simulink model "IEEE9-WT-PV"  (R2024a)
settings: Solver=FixedStepDiscrete  StartTime=0.0  StopTime=Tend  RelTol=1e-3
values from neighbouring files (symbols this model uses):
  beta_0 = 0    [data_WT.m]
  C_4 = 0.1670*C_b    (= 1.00487241952e-06)    [main.m]
  C_6 = 0.2835*C_b    (= 1.70587623314e-06)    [main.m]
  C_8 = 0.2275*C_b    (= 1.36891302659e-06)    [main.m]
  C_dc = 2*S_LV_base*H_DC_base/V_dc_base^2    (= 0.478267523722)    [data_WT.m]    (also in main.m = 1.6)
  C_f = C_f_pu*C_LV_base    (= 0.001461477898)    [data_WT.m]    (also in main.m = 0.00530516476973)
  f_b = 50    [data_WT.m]    (also in main.m)
  fdr_m = 0.05    [main.m]
  fdr_q = 0.01    [main.m]
  G_diff = ss(c2d(s/(20e-3/3*s+1),T_s_cont,'tustin'))    [data_WT.m]
  G_lowpass_disc = ss(c2d(G_lowpass,T_s_cont,'tustin'))    [data_WT.m]
  G_lowpass_disc_1khz = ss(c2d(G_lowpass_1khz,T_s_cont,'tustin'))    [data_WT.m]
  G_setpoint_lowpass_disc = ss(c2d(ss(1/(0.1*s+1)),T_s_cont,'tustin'))    [main.m]
  G_sm_dis = ss(c2d(G_cont_sm,T_s_sim,'tustin'))    [main.m]
  GSC_theta0 = -45.0572/180*pi*0-60/180*pi    (= -1.0471975512)    [data_WT.m]
  I0_total1 = Npar1*I0    (= 7.7895e-08)    [data_PV.m]
  I_GSC_base = S_GSC_base/V_LV_base    (= 30303.030303)    [data_WT.m]
  I_PMSG_0 = T_park(0)^-1*[Z_PMSG^-1*V_LV_base*sqrt(2/3)*([cos(RSC_theta0);sin(RSC_theta0)]-[cos(PMSG_theta0);sin(PMSG_theta0)]);0]    [data_WT.m]
  IL_total1 = Npar1*IL    (= 50459)    [data_PV.m]
  Ipv_scmax1 = Npar1*Ipv_sc    (= 50300)    [data_PV.m]
  island_q = [-0.1312   -0.0230   -0.0343]    [main.m]
  island_Vdc = [1 1.2853    Vpv_mppmax2/Vdc_n]    [main.m]
  island_Vdc_r = [1 1.3430 1.4716]    [main.m]
  island_Vm = [1 1 1]    [main.m]
  J_PMSG_WT_MS = 2*H_PMSGWT_LS*S_PMSG_base/(2*pi*f_b)^2    (= 630.526507942)    [data_WT.m]
  k_p_GSC = 0.02    [data_WT.m]
  k_p_MSC = k_p_GSC    (= 0.02)    [data_WT.m]
  k_theta_GSC = 0.1    [data_WT.m]
  k_theta_MSC = 2/0.6    (= 3.33333333333)    [data_WT.m]
  K_WT_ff_i = 1    [main.m]
  K_WT_ff_v = 1    [main.m]
  K_WT_i_i = 0.79    [main.m]
  K_WT_i_v = 0.69    [main.m]
  K_WT_p_i = 2.1    [main.m]
  K_WT_p_v = 0.15    [main.m]
  Kff_v = 1    [main.m]
  Kffpv_i = 1    [main.m]
  Kp_beta = 270*0    (= 0)    [data_WT.m]
  Kpvi_i1 = Ki_i*Vpv_m/Ipv_b_LV    [main.m]
  Kpvi_v1 = Ki_v*Ipv_b_LV/Vpv_m    [main.m]
  Kpvp_i1 = Kp_i*Vpv_m/Ipv_b_LV    [main.m]
  Kpvp_v1 = Kp_v*Ipv_b_LV/Vpv_m    [main.m]
  L1_pu = 1*0.0186/m    (= 0.000186)    [main.m]
  L_45 = L_lines(2)    [main.m]
  L_56 = L_lines(3)    [main.m]
  L_67 = L_lines(5)    [main.m]
  L_78 = L_lines(6)    [main.m]
  L_89 = L_lines(8)    [main.m]
  L_94 = L_lines(9)    [main.m]
  L_f = L_f_pu*L_LV_base    (= 3.46639466054e-05)    [data_WT.m]    (also in main.m = 9.54929658551e-06)
  L_PMSG = L_PMSG_PU*L_LV_base    (= 3.46639466054e-05)    [data_WT.m]
  main_p = 0.575    [main.m]
  mpv_dc1 = fdr*kg1*w_b/Vdc_n    [main.m]
  mpv_dc1_r = fdr*kg1_r*w_b/Vdc_n    [main.m]
  mpv_p1 = fdr_p/Vdc_n*w_b    [main.m]
  mpv_q1 = fdr_q*Vpv_m/S_b    [main.m]
  Notch_w_10khz = ss(c2d((s^2+w0_f10khz^2)/(s^2+w0_f10khz/Q_f10khz*s+w0_f10khz^2),T_s_sim,'tustin'))    [data_WT.m]
  omega_base = 2*pi*f_b    (= 314.159265359)    [data_WT.m]    (also in main.m)
  omega_wt = 1.4    [data_WT.m]
  R1_pu = 1*0.00734/m    (= 7.34e-05)    [main.m]
  R_45 = R_lines(2)    [main.m]
  R_56 = R_lines(3)    [main.m]
  R_67 = R_lines(5)    [main.m]
  R_78 = R_lines(6)    [main.m]
  R_89 = R_lines(8)    [main.m]
  R_94 = R_lines(9)    [main.m]
  R_f = R_f_pu*Z_LV_base    (= 0.001089)    [data_WT.m]    (also in main.m = 0.0003)
  R_PMSG = R_PMSG_PU*Z_LV_base    (= 0.005445)    [data_WT.m]
  Rpvs_total1 = Rpv_s*Nser1/Npar1    (= 0.0067482)    [data_PV.m]
  RSC_theta0 = 180/180*pi    (= 3.14159265359)    [data_WT.m]
  Rss1 = Vpv_ocmax1/(IL_total1-I0_total1*(exp(Vpv_ocmax1/VT_total1) -1))    [data_PV.m]
  S_b = 100*(10^6)    (= 100000000)    [main.m]
  S_bt = S_b    (= 100000000)    [main.m]
  S_GSC_base = S_LV_base    (= 100000000)    [data_WT.m]
  S_PMSG_base = S_WTPMSG_base    (= 100000000)    [data_WT.m]
  T_load = 20    [main.m]
  T_pitch_servo = 0.5    [data_WT.m]
  T_redispatch = 25    [main.m]
  T_s_cont = 1e-4    (= 0.0001)    [data_WT.m]
  T_s_sim = 1e-7    (= 1e-07)    [data_WT.m]
  V1_rms = 1000    [main.m]
  V2_rms = 13800    [main.m]
  V_dc_base = 7.92e3    (= 7920)    [data_WT.m]
  V_LV_base = 3.3e3    (= 3300)    [data_WT.m]
  V_m = sqrt(2/3)*V1_rms    [main.m]
  v_wind = 12    [data_WT.m]
  Vdc_n = 3*V_m    [main.m]
  Vpv_mppmax1 = Nser1*Vpv_mpp    (= 2945.7)    [data_PV.m]
  Vpv_ocmax1 = Nser1*Vpv_oc    (= 3671.1)    [data_PV.m]
  VT_total1 = VT*Nser1    (= 135.150894483)    [data_PV.m]
  w_b = 2*pi*f_b    (= 314.159265359)    [data_WT.m]    (also in main.m)
undefined symbols (not defined in the file or in its folder): D1, Delta, DiscIntNeverNeededParam, i_dc, PI_pitch
libraries: spsThreePhaseVIMeasurementLib x15, spsThreePhaseSeriesRLCBranchLib x11, spsabctodq0Lib x8, spsThreePhaseTransformerTwoWindingsLib x5, spsThreePhaseParallelRLCLoadLib x5, spsGroundLib x5, spsSeriesRLCBranchLib x5, spsCurrentMeasurementLib x5, spsVoltageMeasurementLib x4, spsPower3phInstantaneousLib x4, spsdq0toabcLib x4, spsThreePhaseParallelRLCBranchLib x3
(part 2 of 3)

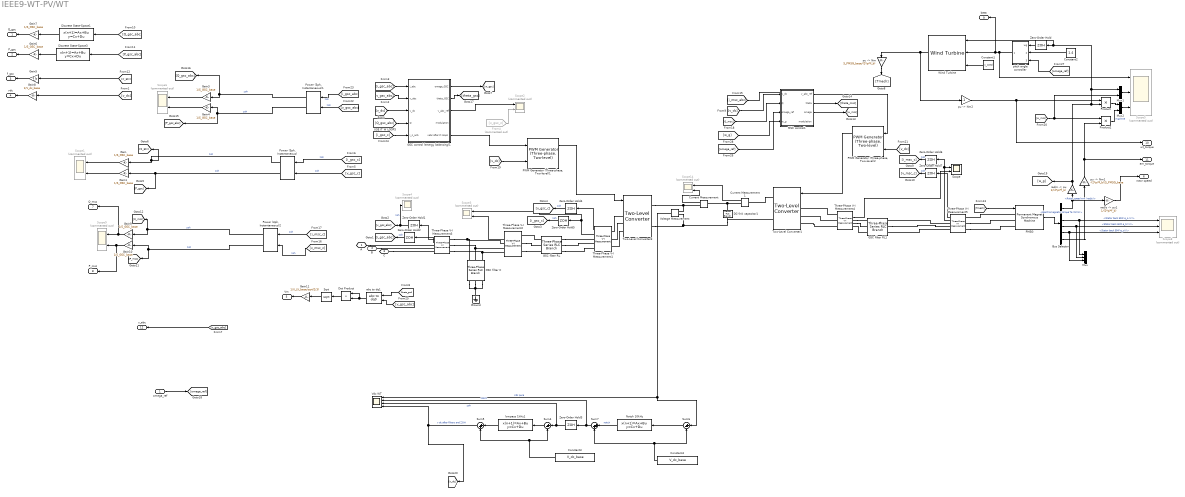
== system IEEE9-WT-PV/WT ==
  omega_ref : Inport
  Bus Selector : BusSelector  OutputSignals=Rotor speed wm (rad/s),Rotor angle thetam (rad),Stator back EMF e_a (V),Stator back EMF e_b (V),Stator back EMF e_cV),Electromagnetic torque Te (N*m)
  Constant1 : Constant  Value=v_wind  SampleTime=T_s_sim
  Constant2 : Constant  Value=1.4  SampleTime=T_s_cont
  Constant3 : Constant  Value=V_dc_base  SampleTime=T_s_cont
  Constant4 : Constant  Value=V_dc_base  SampleTime=T_s_sim
  Current Measurement : spsCurrentMeasurementLib/Current Measurement  PhasorSimulation=off  OutputType=Complex  PSBequivalent=0
  Current Measurement1 : spsCurrentMeasurementLib/Current Measurement  PhasorSimulation=off  OutputType=Complex  PSBequivalent=0
  DC-link capacitor1 : spsSeriesRLCBranchLib/Series RLC Branch  LConnTagsString=__new0  RConnTagsString=__new0  BranchType=C  Resistance=1  Inductance=1e-3  SetiL0=off  InitialCurrent=0  Capacitance=C_dc  Setx0=on  InitialVoltage=V_dc_base  Measurements=None
  Discrete State-Space1 : DiscreteStateSpace  A=G_lowpass_disc.A  B=G_lowpass_disc.B  C=G_lowpass_disc.C  D=G_lowpass_disc.D  SampleTime=T_s_cont
  Discrete State-Space3 : DiscreteStateSpace  A=G_lowpass_disc.A  B=G_lowpass_disc.B  C=G_lowpass_disc.C  D=G_lowpass_disc.D  SampleTime=T_s_cont
  Dot Product : DotProduct  OutDataTypeStr=Inherit: Inherit via internal rule
  From4 : From  Commented=on  GotoTag=v_gsc_c
  GSC control (energy balancing)1 : Subsystem
  GSC filter C : spsThreePhaseSeriesRLCBranchLib/Three-Phase Series RLC Branch  LConnTagsString=A|B|C  RConnTagsString=A|B|C  BranchType=C  Resistance=R_f  Inductance=L_f  Capacitance=C_f  Measurements=None
  GSC filter RL : spsThreePhaseSeriesRLCBranchLib/Three-Phase Series RLC Branch  LConnTagsString=A|B|C  RConnTagsString=A|B|C  BranchType=RL  Resistance=R_f  Inductance=L_f  Capacitance=1e-6  Measurements=None
  GSC filter RL1 : spsThreePhaseSeriesRLCBranchLib/Three-Phase Series RLC Branch  LConnTagsString=A|B|C  RConnTagsString=A|B|C  BranchType=RL  Resistance=R_f  Inductance=L_f  Capacitance=1e-6  Measurements=None
  Gain{,1,3..4,6..7,9..10} (8 alike) : Gain  Gain=1/S_GSC_base
  Gain11 : Gain  Gain=1/V_LV_base/sqrt(2/3)
  Gain5 : Gain  Gain=f_b
  Gain8 : Gain  Gain=1/V_dc_base
  Ground : spsGroundLib/Ground  LConnTagsString=a
  MSC control1 : Subsystem
  Mux : Mux  Inputs=3
  Mux1 : Mux  Inputs=2
  Mux2 : Mux  Inputs=2
  Notch 10kHz : DiscreteStateSpace  A=Notch_w_10khz.A  B=Notch_w_10khz.B  C=Notch_w_10khz.C  D=Notch_w_10khz.D  SampleTime=T_s_sim
  PMSG : spsPermanentMagnetSynchronousMachineLib/Permanent Magnet Synchronous Machine  NbPhases=3  FluxDistribution=Trapezoidal  RotorType=Round  MechanicalLoad=Torque Tm  PresetModel=No  ShowDetailedParameters=on  MeasurementBus=off  Resistance=R_PMSG  Inductance=L_PMSG  dqInductances=[8.5e-3,8.5e-3]  La=L_PMSG  MachineConstant=Flux linkage established by magnets (V.s)  Flux=V_LV_base/(omega_wt*f_b*2*pi)*sqrt(2/3)*1  VoltageCst=1111.1678  TorqueCst=10.6109  Flat=0  Mechanical=[J_PMSG_WT_MS 0.001 1 0]  PolePairs=1  InitialConditions=[omega_wt*f_b*2*pi,0, I_PMSG_0(1),I_PMSG_0(2)]  InitialConditions5ph=[0 0 0 0 0 0]  RefAngle=Aligned with phase A axis (original Park)  IterativeDiscreteModel=Backward Euler robust  TsBlock=T_s_sim  TsPowergui=0
  "PWM Generator (Three-phase, Two-level)1" : eePwmGeneratorTwoLevel/PWM Generator (Three-phase, Two-level)  PWMMode=Continuous PWM (CPWM)  CPWMMode=SPWM: sinusoidal PWM  DPWMMode=60 DPWM: 60 degree discontinuous PWM  fsw=10e3  Ts=T_s_sim
  "PWM Generator (Three-phase, Two-level)2" : eePwmGeneratorTwoLevel/PWM Generator (Three-phase, Two-level)  PWMMode=Continuous PWM (CPWM)  CPWMMode=SPWM: sinusoidal PWM  DPWMMode=60 DPWM: 60 degree discontinuous PWM  fsw=10e3  Ts=T_s_sim
  "Power (3ph, Instantaneous)" : spsPower3phInstantaneousLib/Power (3ph, Instantaneous)
  "Power (3ph, Instantaneous)1" : spsPower3phInstantaneousLib/Power (3ph, Instantaneous)
  "Power (3ph, Instantaneous)2" : spsPower3phInstantaneousLib/Power (3ph, Instantaneous)
  Product : Product
  Product1 : Product
  Scope : Scope  NumInputPorts=2
  Scope{1..3,6,9,14} (6 alike) : Scope  Commented=on  NumInputPorts=2
  Scope4 : Scope  Commented=on
  Scope5 : Scope  Commented=on  NumInputPorts=3
  Scope8 : Scope  Commented=on  NumInputPorts=3
  Sqrt : Sqrt
  Sum4 : Sum  Inputs=|+-
  Sum5 : Sum  Inputs=|++
  Sum6 : Sum  Inputs=|+-
  Sum7 : Sum  Inputs=|++
  Three-Phase V-I Measurement{1..5} (5 alike) : spsThreePhaseVIMeasurementLib/Three-Phase V-I Measurement  VoltageMeasurement=phase-to-ground  SetLabelV=off  LabelV=Vabc  Vpu=off  VpuLL=off  CurrentMeasurement=yes  SetLabelI=off  LabelI=Iabc  Ipu=off  Pbase=100e6  Vbase=500e3  OutputType=Complex  PhasorSimulation=off  PSBequivalent=0
  Two-Level Converter1 : spsTwoLevelConverterLib/Two-Level Converter  ModelType=Switching devices  Ron=1e-3  Rs=1e6  Cs=inf  Vforward=[0,0]  Ron_Diode=1e-3  Rs_Diode=1e6  Cs_Diode=inf  Vf_Diode=1e-3  Rs_CurrentSource=inf  Ron_ACsource=1e-3
  Two-Level Converter3 : spsTwoLevelConverterLib/Two-Level Converter  ModelType=Switching devices  Ron=1e-3  Rs=1e6  Cs=inf  Vforward=[0,0]  Ron_Diode=1e-3  Rs_Diode=1e6  Cs_Diode=inf  Vf_Diode=1e-3  Rs_CurrentSource=inf  Ron_ACsource=1e-3
  Vdc WT : Scope  NumInputPorts=4
  Voltage Measurement : spsVoltageMeasurementLib/Voltage Measurement  PhasorSimulation=off  OutputType=Complex  PSBequivalent=0
  Wind Turbine : spsWindTurbineLib/Wind Turbine  Pnom=S_PMSG_base  Pelec_base=S_PMSG_base  wind_base=12  P_wind_base=0.75  speed_nom=1.2  pitch_angle=beta_0  c1_c6="[0.51763          116          0.4            5           21     0.006795]"  cp_nom=0.48  lambda_nom=8.1
  Zero-Order Hold{,1..7} (8 alike) : ZeroOrderHold  SampleTime=T_s_cont
  abc to dq1 : spsabctodq0Lib/abc to dq0  Alignment=90 degrees behind phase A axis
  lowpass 1kHz1 : DiscreteStateSpace  A=G_lowpass_disc_1khz.A  B=G_lowpass_disc_1khz.B  C=G_lowpass_disc_1khz.C  D=G_lowpass_disc_1khz.D  SampleTime=T_s_cont
  pitch angle controller : Subsystem
  "pu -> Nm" : Gain  Gain=S_PMSG_base/(2*pi*f_b)
  "pu -> Nm1" : Gain  Gain=-(2*pi*f_b)/S_PMSG_base
  "pu -> Nm2" : Gain  Gain=-1
  "rad/s -> pu" : Gain  Gain=1/(2*pi*f_b)
  "rad/s -> pu1" : Gain  Gain=1/(2*pi*f_b)
  A : PMIOPort  Side=Right
  B : PMIOPort  Port=2  Side=Right
  C : PMIOPort  Port=3  Side=Right
  Q_gsc : Outport
  P_gsc : Outport  Port=2
  f_gsc : Outport  Port=3
  vdc : Outport  Port=4
  Vm : Outport  Port=5
  rotor speed : Outport  Port=6
  Q_msc : Outport  Port=7
  P_msc : Outport  Port=8
  beta : Outport  Port=9
  wt_torque : Outport  Port=10
  em_torque : Outport  Port=11
  v_abc : Outport  Port=12  VectorParamsAs1DForOutWhenUnconnected=off
  wires:
  Wind Turbine/1 -> "pu -> Nm"/1, "pu -> Nm2"/1
  "rad/s -> pu"/1 -> Wind Turbine/1, Zero-Order Hold/1, Mux1/1, Product/2, [w_g]
  Constant1/1 -> Wind Turbine/3
  GSC control (energy balancing)1/3(v_abc_ref) -> Scope2/1
  Bus Selector/1 -> "rad/s -> pu1"/1, "rad/s -> pu"/1  "<Rotor speed wm (rad/s)>"
  GSC control (energy balancing)1/1(omega_GSC) -> [w_gsc]
  Bus Selector/4 -> Mux/2, Scope8/2  "<Stator back EMF e_b (V)>"
  Bus Selector/3 -> Mux/1, Scope8/1  "<Stator back EMF e_a (V)>"
  Bus Selector/5 -> Mux/3, Scope8/3  "<Stator back EMF e_cV)>"
  Gain1/1 -> Scope1/2
  Gain/1 -> Scope1/1
  PMSG/1 -> Bus Selector/1
  Constant2/1 -> pitch angle controller/2(max)
  pitch angle controller/1(pitch) -> Scope5/1, Wind Turbine/2, beta/1
  Mux1/1 -> Scope5/2
  Mux2/1 -> Scope5/3
  Product/1 -> Mux2/1
  Bus Selector/6 -> "pu -> Nm1"/1  "<Electromagnetic torque Te (N*m)>"
  Product1/1 -> Mux2/2  "machine"
  "pu -> Nm1"/1 -> em_torque/1, Product1/2
  Gain5/1 -> f_gsc/1
  [v_dc] -> GSC control (energy balancing)1/3(v_dc)
  [v_dc] -> Gain8/1
  Three-Phase V-I Measurement3/1 -> Zero-Order Hold1/1
  [v_gsc_abc] -> GSC control (energy balancing)1/2(v_abc)
  [i_gsc_abc] -> GSC control (energy balancing)1/1(i_abc)
  Three-Phase V-I Measurement1/2 -> Scope3/1, Zero-Order Hold5/1
  Three-Phase V-I Measurement1/1 -> Zero-Order Hold4/1
  From4/1 -> Scope2/2
  [v_dc] -> MSC control1/1(v_dc)
  [Q_gsc_abc] -> Discrete State-Space1/1
  [P_gsc_abc] -> Discrete State-Space3/1
  Gain6/1 -> P_gsc/1
  Gain7/1 -> Q_gsc/1
  Gain8/1 -> vdc/1
  [w_gsc] -> Gain5/1
  "pu -> Nm"/1 -> [Tmech]
  [Tmech] -> PMSG/1
  [i_msc_abc] -> ?
  Gain9/1 -> Q_msc/1, Scope9/1
  Gain10/1 -> P_msc/1, Scope9/2
  MSC control1/3(omega) -> [w_msc]
  [w_msc] -> Mux1/2, Product1/1
  MSC control1/2(theta) -> [theta_msc]
  Gain4/1 -> Scope6/2
  Gain3/1 -> Scope6/1
  Three-Phase V-I Measurement3/2 -> Zero-Order Hold2/1
  Zero-Order Hold/1 -> pitch angle controller/1(wg)
  [i_gsc_c] -> GSC control (energy balancing)1/5(i_s_acb)
  [Q_gsc_abc] -> GSC control (energy balancing)1/4(Q)
  GSC control (energy balancing)1/2(theta_GSC) -> [theta_gsc]
  Current Measurement1/1 -> Scope14/1
  Current Measurement/1 -> Scope14/2
  [theta_gsc] -> abc to dq1/2
  [v_gsc_abc] -> abc to dq1/1
  abc to dq1/1 -> Dot Product/1, Dot Product/2
  Dot Product/1 -> Sqrt/1
  Gain11/1 -> Vm/1
  Sqrt/1 -> Gain11/1
  "rad/s -> pu1"/1 -> rotor speed/1
  "pu -> Nm2"/1 -> wt_torque/1, Product/1
  omega_ref/1 -> [omega_ref]
  [omega_ref] -> MSC control1/3(omega_ref)
  [omega_ref] -> pitch angle controller/3(omega_ref)
  [w_g] -> MSC control1/4(w_g)
  [Q_msc] -> MSC control1/2(Q)
  Three-Phase V-I Measurement5/2 -> Zero-Order Hold6/1, Scope/1
  Constant4/1 -> Sum6/2, Sum7/2
  Notch 10kHz/1 -> Sum7/1  "notch"
  Voltage Measurement/1 -> Sum6/1, Vdc WT/1  "Vdc pure"
  Sum4/1 -> lowpass 1kHz1/1
  lowpass 1kHz1/1 -> Sum5/1
  Sum7/1 -> Zero-Order Hold3/1, Vdc WT/2  "notch"
  Sum6/1 -> Notch 10kHz/1
  Constant3/1 -> Sum4/2, Sum5/2
  GSC control (energy balancing)1/5(vabc after PI loops) -> "PWM Generator (Three-phase, Two-level)1"/1
  [v_dc] -> "PWM Generator (Three-phase, Two-level)1"/2
  [v_dc] -> "PWM Generator (Three-phase, Two-level)2"/2
  [i_msc_c] -> "Power (3ph, Instantaneous)2"/2  "zoh"
  [v_msc_c] -> "Power (3ph, Instantaneous)2"/1  "zoh"
  [v_gsc_c] -> "Power (3ph, Instantaneous)"/1  "zoh"
  [i_gsc_c] -> "Power (3ph, Instantaneous)"/2  "zoh"
  [v_gsc_abc] -> "Power (3ph, Instantaneous)1"/1  "zoh"
  [i_gsc_abc] -> "Power (3ph, Instantaneous)1"/2  "zoh"
  MSC control1/1(v_abc_ref) -> "PWM Generator (Three-phase, Two-level)2"/1
  Three-Phase V-I Measurement5/1 -> Zero-Order Hold7/1
  Three-Phase V-I Measurement4/2 -> Scope/2
  Three-Phase V-I Measurement2/2 -> Scope3/2
  Sum5/1 -> [v_dc], Vdc WT/4  "v dc after filters and ZOH"
  "Power (3ph, Instantaneous)2"/2 -> Gain9/1, [Q_msc]  "zoh"
  "Power (3ph, Instantaneous)2"/1 -> Gain10/1, [P_msc]  "zoh"
  "Power (3ph, Instantaneous)1"/2 -> Gain3/1, [Q_gsc_abc]  "zoh"
  "Power (3ph, Instantaneous)1"/1 -> Gain4/1, [P_gsc_abc]  "zoh"
  "Power (3ph, Instantaneous)"/2 -> Gain/1, [Q_gsc]  "zoh"
  "Power (3ph, Instantaneous)"/1 -> [P_gsc], Gain1/1  "zoh"
  Zero-Order Hold3/1 -> Sum4/1, Vdc WT/3  "zoh"
  "PWM Generator (Three-phase, Two-level)2"/1 -> Two-Level Converter1/1
  Discrete State-Space1/1 -> Gain7/1
  Discrete State-Space3/1 -> Gain6/1
  "PWM Generator (Three-phase, Two-level)1"/1 -> Two-Level Converter3/1
  Zero-Order Hold1/1 -> Scope4/1, [v_gsc_abc]  "zoh"
  Zero-Order Hold2/1 -> [i_gsc_abc]  "zoh"
  Zero-Order Hold4/1 -> [v_gsc_c]  "zoh"
  Zero-Order Hold5/1 -> [i_gsc_c]  "zoh"
  Zero-Order Hold6/1 -> [i_msc_c]  "zoh"
  Zero-Order Hold7/1 -> [v_msc_c]  "zoh"
  [v_gsc_abc] -> v_abc/1
  connections:
  DC-link capacitor1/LConn1 -- Current Measurement/LConn1 -- Current Measurement1/RConn1
  GSC filter C/RConn3 -- GSC filter C/RConn1 -- GSC filter C/RConn2 -- Ground/LConn1
  Voltage Measurement/LConn2 -- Two-Level Converter3/RConn2 -- Two-Level Converter1/RConn2 -- DC-link capacitor1/RConn1
  Current Measurement/RConn1 -- Voltage Measurement/LConn1 -- Two-Level Converter3/RConn1
  Three-Phase V-I Measurement5/RConn1 -- GSC filter RL1/RConn1
  Three-Phase V-I Measurement5/RConn3 -- GSC filter RL1/RConn3
  Three-Phase V-I Measurement5/LConn2 -- PMSG/LConn2
  Two-Level Converter1/RConn1 -- Current Measurement1/LConn1
  Two-Level Converter3/LConn2 -- Three-Phase V-I Measurement1/LConn2
  Two-Level Converter3/LConn3 -- Three-Phase V-I Measurement1/LConn3
  Three-Phase V-I Measurement3/LConn1 -- Three-Phase V-I Measurement2/RConn1 -- GSC filter C/LConn1
  Three-Phase V-I Measurement3/LConn3 -- Three-Phase V-I Measurement2/RConn3 -- GSC filter C/LConn3
  Three-Phase V-I Measurement3/LConn2 -- Three-Phase V-I Measurement2/RConn2 -- GSC filter C/LConn2
  Two-Level Converter3/LConn1 -- Three-Phase V-I Measurement1/LConn1
  Three-Phase V-I Measurement5/LConn3 -- PMSG/LConn3
  A/RConn1 -- Three-Phase V-I Measurement3/RConn1
  B/RConn1 -- Three-Phase V-I Measurement3/RConn2
  C/RConn1 -- Three-Phase V-I Measurement3/RConn3
  Three-Phase V-I Measurement4/LConn1 -- Two-Level Converter1/LConn1
  Three-Phase V-I Measurement4/LConn2 -- Two-Level Converter1/LConn2
  Three-Phase V-I Measurement4/RConn2 -- GSC filter RL1/LConn2
  Three-Phase V-I Measurement4/RConn1 -- GSC filter RL1/LConn1
  GSC filter RL/RConn1 -- Three-Phase V-I Measurement1/RConn1
  GSC filter RL/RConn2 -- Three-Phase V-I Measurement1/RConn2
  GSC filter RL/RConn3 -- Three-Phase V-I Measurement1/RConn3
  Three-Phase V-I Measurement4/LConn3 -- Two-Level Converter1/LConn3
  GSC filter RL1/LConn3 -- Three-Phase V-I Measurement4/RConn3
  GSC filter RL1/RConn2 -- Three-Phase V-I Measurement5/RConn2
  PMSG/LConn1 -- Three-Phase V-I Measurement5/LConn1
  Three-Phase V-I Measurement2/LConn3 -- GSC filter RL/LConn3
  Three-Phase V-I Measurement2/LConn2 -- GSC filter RL/LConn2
  GSC filter RL/LConn1 -- Three-Phase V-I Measurement2/LConn1

== system IEEE9-WT-PV/Synchronous Machine/Subsystem2 ==
  P_ref : Inport
  speed_ref : Inport  Port=2
  speed : Inport  Port=3
  1/droop : Gain  Gain=1/fdr_m
  Delta load setpoint : Sum  Inputs=+-|
  Delta speed : Sum  Inputs=-+|
  throttle : Outport  VectorParamsAs1DForOutWhenUnconnected=off
  wires:
  speed/1 -> Delta speed/2
  1/droop/1 -> Delta load setpoint/2
  Delta speed/1 -> 1/droop/1
  speed_ref/1 -> Delta speed/1
  P_ref/1 -> Delta load setpoint/1
  Delta load setpoint/1 -> throttle/1

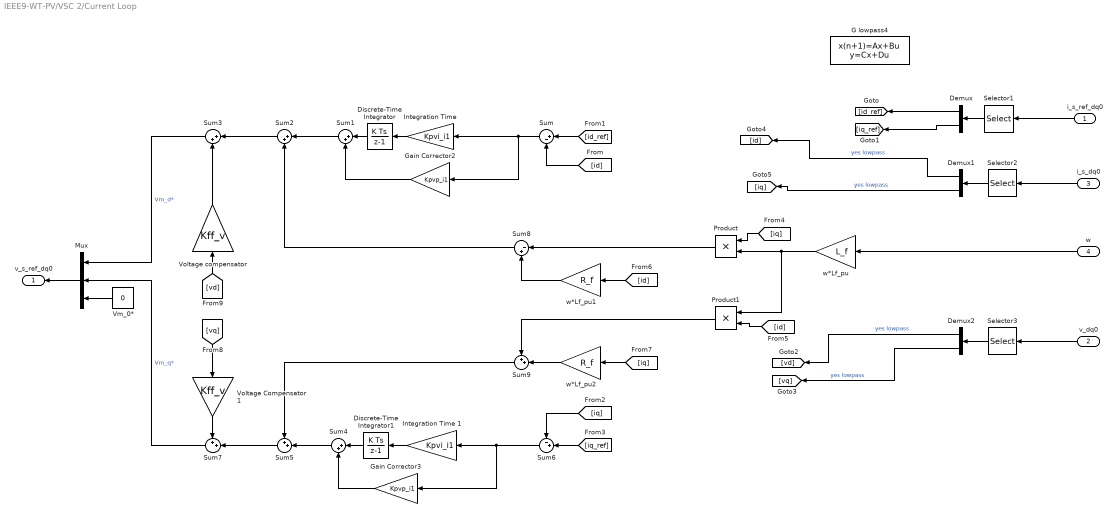
== system IEEE9-WT-PV/VSC 2/Current Loop ==
  i_s_ref_dq0 : Inport
  v_dq0 : Inport  Port=2
  i_s_dq0 : Inport  Port=3
  w : Inport  Port=4
  Demux : Demux  Outputs=2
  Demux1 : Demux  Outputs=2
  Demux2 : Demux  Outputs=2
  Discrete-Time Integrator : DiscreteIntegrator  SampleTime=T_s_cont  ICPrevOutput=DiscIntNeverNeededParam  ICPrevScaledInput=DiscIntNeverNeededParam
  Discrete-Time Integrator1 : DiscreteIntegrator  SampleTime=T_s_cont  ICPrevOutput=DiscIntNeverNeededParam  ICPrevScaledInput=DiscIntNeverNeededParam
  G lowpass4 : DiscreteStateSpace  A=G_lowpass_disc_1khz.A  B=G_lowpass_disc_1khz.B  C=G_lowpass_disc_1khz.C  D=G_lowpass_disc_1khz.D  SampleTime=T_s_cont
  Gain Corrector2 : Gain  Gain=Kpvp_i1
  Gain Corrector3 : Gain  Gain=Kpvp_i1
  Integration Time : Gain  Gain=Kpvi_i1
  Integration Time 1 : Gain  Gain=Kpvi_i1
  Mux : Mux  Inputs=3
  Product : Product  RndMeth=Zero
  Product1 : Product  RndMeth=Zero
  Selector1 : Selector  InputPortWidth=3  IndexOptions=Index vector (dialog)  Indices=[1 2]  OutputSizes=1
  Selector2 : Selector  InputPortWidth=3  IndexOptions=Index vector (dialog)  Indices=[1 2]  OutputSizes=1
  Selector3 : Selector  InputPortWidth=3  IndexOptions=Index vector (dialog)  Indices=[1 2]  OutputSizes=1
  Sum : Sum  Inputs=|+-
  Sum{1..4} (4 alike) : Sum  Inputs=|++
  Sum5 : Sum  Inputs=++|
  Sum6 : Sum  Inputs=-+|
  Sum7 : Sum  Inputs=++|
  Sum8 : Sum  Inputs=|-+
  Sum9 : Sum  Inputs=++|
  Vm_0* : Constant  Value=0  SampleTime=T_s_cont
  Voltage Compensator 1 : Gain  Gain=Kff_v
  Voltage compensator : Gain  Gain=Kff_v
  w*Lf_pu : Gain  Gain=L_f
  w*Lf_pu1 : Gain  Gain=R_f
  w*Lf_pu2 : Gain  Gain=R_f
  v_s_ref_dq0 : Outport  VectorParamsAs1DForOutWhenUnconnected=off
  wires:
  Integration Time 1/1 -> Discrete-Time Integrator1/1
  Integration Time/1 -> Discrete-Time Integrator/1
  Sum5/1 -> Sum7/2
  Sum3/1 -> Mux/1  "Vm_d*"
  Sum7/1 -> Mux/2  "Vm_q*"
  Voltage Compensator 1/1 -> Sum7/1
  w*Lf_pu/1 -> Product1/1, Product/2
  i_s_ref_dq0/1 -> Selector1/1
  Discrete-Time Integrator1/1 -> Sum4/1
  Voltage compensator/1 -> Sum3/2
  Sum2/1 -> Sum3/1
  Selector1/1 -> Demux/1
  Sum1/1 -> Sum2/1
  w/1 -> w*Lf_pu/1
  Mux/1 -> v_s_ref_dq0/1
  Selector2/1 -> Demux1/1
  Selector3/1 -> Demux2/1
  Vm_0*/1 -> Mux/3
  Discrete-Time Integrator/1 -> Sum1/1
  Sum4/1 -> Sum5/2
  Sum/1 -> Integration Time/1, Gain Corrector2/1
  Sum6/1 -> Integration Time 1/1, Gain Corrector3/1
  Demux/1 -> [id_ref]
  Demux/2 -> [iq_ref]
  [id] -> Sum/2
  [id_ref] -> Sum/1
  [iq_ref] -> Sum6/2
  [iq] -> Sum6/1
  Gain Corrector2/1 -> Sum1/2
  Gain Corrector3/1 -> Sum4/2
  [iq] -> Product/1
  [id] -> Product1/2
  Product/1 -> Sum8/1
  [id] -> w*Lf_pu1/1
  w*Lf_pu1/1 -> Sum8/2
  Sum8/1 -> Sum2/2
  Product1/1 -> Sum9/1
  [iq] -> w*Lf_pu2/1
  w*Lf_pu2/1 -> Sum9/2
  Sum9/1 -> Sum5/1
  [vq] -> Voltage Compensator 1/1
  [vd] -> Voltage compensator/1
  v_dq0/1 -> Selector3/1
  i_s_dq0/1 -> Selector2/1
  Demux2/2 -> [vq]  "yes lowpass"
  Demux1/2 -> [iq]  "yes lowpass"
  Demux1/1 -> [id]  "yes lowpass"
  Demux2/1 -> [vd]  "yes lowpass"

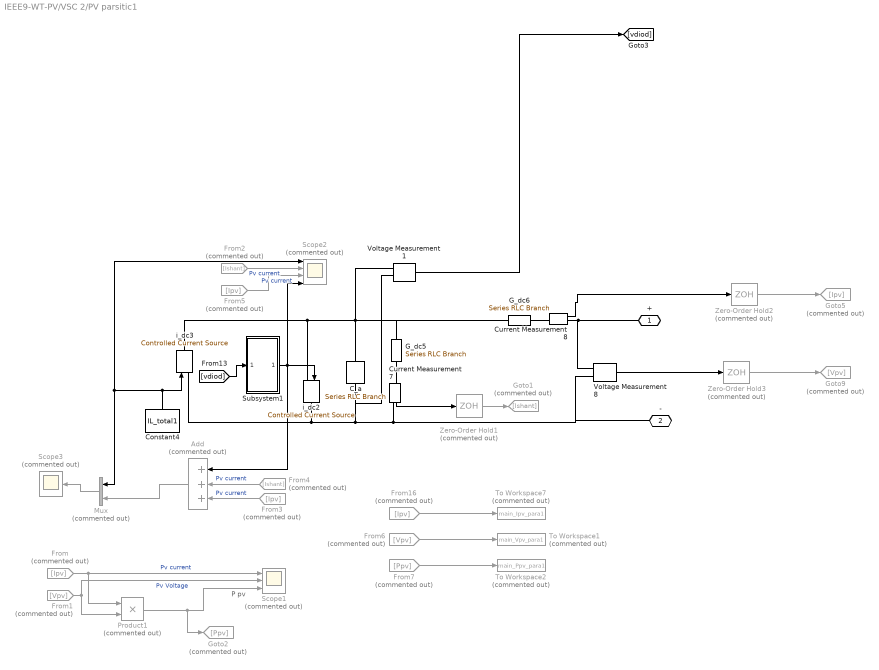
== system IEEE9-WT-PV/VSC 2/PV parsitic1 ==
  note: P pv
  Add : Sum  Commented=on  Inputs=+++
  C_a : spsSeriesRLCBranchLib/Series RLC Branch  LConnTagsString=__new0  RConnTagsString=__new0  BranchType=C  Resistance=1  Inductance=1e-3  SetiL0=off  InitialCurrent=0  Capacitance=75e-12  Setx0=on  InitialVoltage=island_Vdc(2)*Vdc_n  Measurements=None
  Constant4 : Constant  Value=IL_total1  SampleTime=T_s_sim
  Current Measurement7 : spsCurrentMeasurementLib/Current Measurement  PhasorSimulation=off  OutputType=Complex  PSBequivalent=0
  Current Measurement8 : spsCurrentMeasurementLib/Current Measurement  PhasorSimulation=off  OutputType=Complex  PSBequivalent=0
  From{,3,5,16} (4 alike) : From  Commented=on  GotoTag=Ipv
  From1 : From  Commented=on  GotoTag=Vpv
  From2 : From  Commented=on  GotoTag=Ishant
  From4 : From  Commented=on  GotoTag=Ishant
  From6 : From  Commented=on  GotoTag=Vpv
  From7 : From  Commented=on  GotoTag=Ppv
  G_dc5 : spsSeriesRLCBranchLib/Series RLC Branch  LConnTagsString=__new0  RConnTagsString=__new0  BranchType=R  Resistance=Rss1  Inductance=1e-3  SetiL0=off  InitialCurrent=0  Capacitance=1e-6  Setx0=off  InitialVoltage=0  Measurements=None
  G_dc6 : spsSeriesRLCBranchLib/Series RLC Branch  LConnTagsString=__new0  RConnTagsString=__new0  BranchType=R  Resistance=Rpvs_total1  Inductance=1e-3  SetiL0=off  InitialCurrent=0  Capacitance=1e-6  Setx0=off  InitialVoltage=0  Measurements=None
  Goto1 : Goto  Commented=on  GotoTag=Ishant
  Goto2 : Goto  Commented=on  GotoTag=Ppv
  Goto5 : Goto  Commented=on  GotoTag=Ipv
  Goto9 : Goto  Commented=on  GotoTag=Vpv
  Mux : Mux  Commented=on  Inputs=2
  Product1 : Product  Commented=on
  Scope1 : Scope  Commented=on  NumInputPorts=3
  Scope2 : Scope  Commented=on  NumInputPorts=4
  Scope3 : Scope  Commented=on
  Subsystem1 : Subsystem
  To Workspace1 : ToWorkspace  Commented=on  VariableName=main_Vpv_para1  SampleTime=-1
  To Workspace2 : ToWorkspace  Commented=on  VariableName=main_Ppv_para1  SampleTime=-1
  To Workspace7 : ToWorkspace  Commented=on  VariableName=main_Ipv_para1  SampleTime=-1
  Voltage Measurement1 : spsVoltageMeasurementLib/Voltage Measurement  PhasorSimulation=off  OutputType=Complex  PSBequivalent=0
  Voltage Measurement8 : spsVoltageMeasurementLib/Voltage Measurement  PhasorSimulation=off  OutputType=Complex  PSBequivalent=0
  Zero-Order Hold1 : ZeroOrderHold  Commented=on  SampleTime=T_s_sim
  Zero-Order Hold2 : ZeroOrderHold  Commented=on  SampleTime=T_s_sim
  Zero-Order Hold3 : ZeroOrderHold  Commented=on  SampleTime=T_s_sim
  i_dc2 : spsControlledCurrentSourceLib/Controlled Current Source  Initialize=off  Source_Type=DC  Amplitude=i_dc  Phase=0  Frequency=0  Measurements=None
  i_dc3 : spsControlledCurrentSourceLib/Controlled Current Source  Initialize=off  Source_Type=DC  Amplitude=i_dc  Phase=0  Frequency=0  Measurements=None
  + : PMIOPort  Side=Right
  - : PMIOPort  Port=2  Side=Right
  wires:
  Voltage Measurement8/1 -> Zero-Order Hold3/1
  Current Measurement8/1 -> Zero-Order Hold2/1
  From7/1 -> To Workspace2/1
  From6/1 -> To Workspace1/1
  From16/1 -> To Workspace7/1
  From2/1 -> Scope2/2  "Pv current"
  From4/1 -> Add/2  "Pv current"
  Add/1 -> Mux/2
  [vdiod] -> Subsystem1/1(Vpv)
  Constant4/1 -> i_dc3/1, Scope2/1, Mux/1
  Product1/1 -> Scope1/3, Goto2/1
  Subsystem1/1(Idiod) -> Add/1, i_dc2/1, Scope2/4
  From5/1 -> Scope2/3  "Pv current"
  Mux/1 -> Scope3/1
  From/1 -> Product1/1, Scope1/1  "Pv current"
  From1/1 -> Scope1/2, Product1/2  "Pv Voltage"
  From3/1 -> Add/3  "Pv current"
  Current Measurement7/1 -> Zero-Order Hold1/1
  Zero-Order Hold1/1 -> Goto1/1
  Zero-Order Hold2/1 -> Goto5/1
  Zero-Order Hold3/1 -> Goto9/1
  Voltage Measurement1/1 -> [vdiod]
  connections:
  Current Measurement8/LConn1 -- G_dc6/RConn1
  Current Measurement7/LConn1 -- G_dc5/RConn1
  Current Measurement8/RConn1 -- Voltage Measurement8/LConn1 -- +/RConn1
  C_a/LConn1 -- i_dc3/RConn1 -- i_dc2/LConn1 -- G_dc6/LConn1 -- G_dc5/LConn1 -- Voltage Measurement1/LConn1
  i_dc2/RConn1 -- i_dc3/LConn1 -- Current Measurement7/RConn1 -- -/RConn1 -- Voltage Measurement8/LConn2 -- C_a/RConn1 -- Voltage Measurement1/LConn2

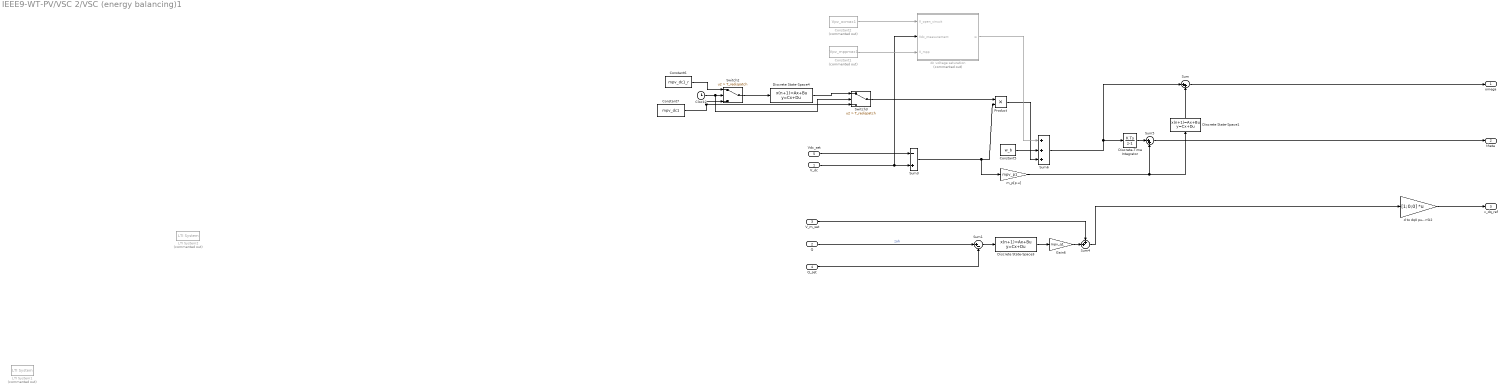
== system IEEE9-WT-PV/VSC 2/VSC (energy balancing)1 ==
  V_dc : Inport
  Q : Inport  Port=2
  V_m_set : Inport  Port=3
  Q_set : Inport  Port=4
  Vdc_set : Inport  Port=5
  Clock2 : Clock
  Constant1 : Constant  Commented=on  Value=Vpv_mppmax1  SampleTime=T_s_cont
  Constant2 : Constant  Commented=on  Value=Vpv_ocmax1  SampleTime=T_s_cont
  Constant5 : Constant  Value=w_b  SampleTime=T_s_cont
  Constant6 : Constant  Value=mpv_dc1_r  SampleTime=T_s_cont
  Constant7 : Constant  Value=mpv_dc1  SampleTime=T_s_cont
  Discrete State-Space1 : DiscreteStateSpace  A=G_diff.A  B=G_diff.B  C=G_diff.C  D=G_diff.D  SampleTime=T_s_cont
  Discrete State-Space3 : DiscreteStateSpace  A=G_lowpass_disc.A  B=G_lowpass_disc.B  C=G_lowpass_disc.C  D=G_lowpass_disc.D  SampleTime=T_s_cont
  Discrete State-Space4 : DiscreteStateSpace  A=G_setpoint_lowpass_disc.A  B=G_setpoint_lowpass_disc.B  C=G_setpoint_lowpass_disc.C  D=G_setpoint_lowpass_disc.D  SampleTime=T_s_cont
  Discrete-Time Integrator : DiscreteIntegrator  SampleTime=T_s_cont  ICPrevOutput=DiscIntNeverNeededParam  ICPrevScaledInput=DiscIntNeverNeededParam
  Gain6 : Gain  Gain=mpv_q1
  LTI System1 : cstblocks/LTI System  Commented=on  sys=G_lp_d  IC=[]  PadeOrder=0
  LTI System2 : cstblocks/LTI System  Commented=on  sys=G_dif_c  IC=[]  PadeOrder=0
  Product : Product
  Sum : Sum  Inputs=|++
  Sum1 : Sum  Inputs=|+-
  Sum3 : Sum  Inputs=-+
  Sum4 : Sum  Inputs=++|
  Sum5 : Sum  Inputs=|++
  Sum6 : Sum  Inputs=+++
  Switch2 : Switch  Criteria=u2 > Threshold  Threshold=T_redispatch  SaturateOnIntegerOverflow=off  InputSameDT=off
  Switch3 : Switch  Criteria=u2 > Threshold  Threshold=T_redispatch  SaturateOnIntegerOverflow=off  InputSameDT=off
  d to dq0 pu-->SI2 : Gain  Gain=[1;0;0]  Multiplication=Matrix(K*u) (u vector)
  dc voltage saturation : Subsystem  Commented=on
  m_p[p.u] : Gain  Gain=mpv_p1
  omega : Outport
  theta : Outport  Port=2
  v_dq_ref : Outport  Port=3
  wires:
  Discrete-Time Integrator/1 -> Sum5/1
  m_p[p.u]/1 -> Discrete State-Space1/1, Sum5/2
  Sum6/1 -> Sum/1, Discrete-Time Integrator/1
  Discrete State-Space1/1 -> Sum/2
  Gain6/1 -> Sum4/2
  Q_set/1 -> Sum1/2
  V_m_set/1 -> Sum4/1
  Sum/1 -> omega/1
  Sum5/1 -> theta/1
  Sum4/1 -> d to dq0 pu-->SI2/1
  Vdc_set/1 -> Sum3/1
  d to dq0 pu-->SI2/1 -> v_dq_ref/1
  Constant5/1 -> Sum6/2
  Constant2/1 -> dc voltage saturation/1(V_open_circuit)
  V_dc/1 -> dc voltage saturation/2(Vdc_measurement), Sum3/2
  Constant1/1 -> dc voltage saturation/3(V_mpp)
  Sum1/1 -> Discrete State-Space3/1
  Discrete State-Space4/1 -> Switch3/1
  Clock2/1 -> Switch3/2, Switch2/2
  Constant6/1 -> Switch2/1
  Switch2/1 -> Discrete State-Space4/1
  Constant7/1 -> Switch2/3, Switch3/3
  Switch3/1 -> Product/1
  Product/1 -> Sum6/3
  Discrete State-Space3/1 -> Gain6/1
  Q/1 -> Sum1/1  "zoh"
  Sum3/1 -> Product/2, m_p[p.u]/1
  dc voltage saturation/1(w) -> Sum6/1

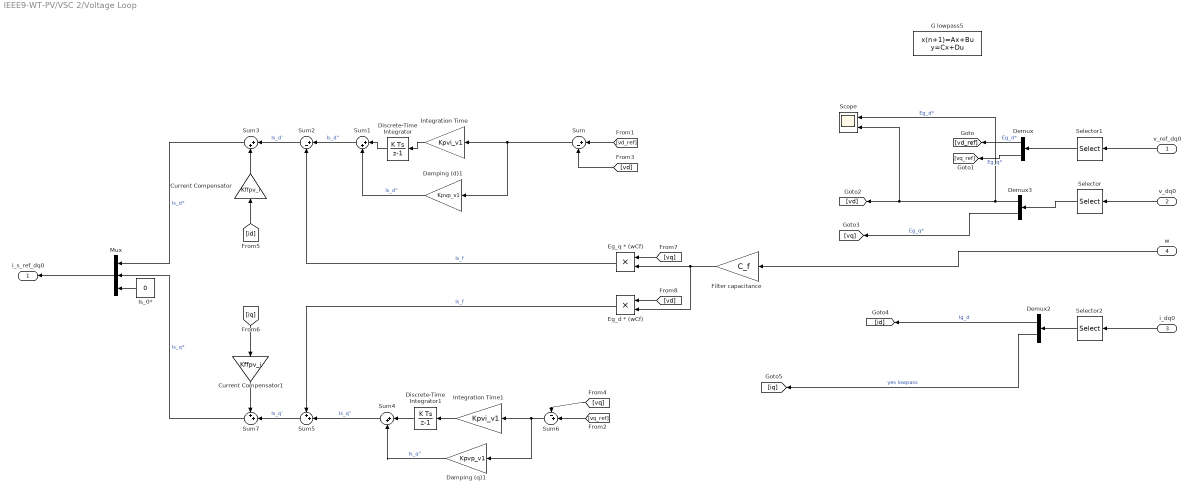
== system IEEE9-WT-PV/VSC 2/Voltage Loop ==
  v_ref_dq0 : Inport
  v_dq0 : Inport  Port=2
  i_dq0 : Inport  Port=3
  w : Inport  Port=4
  Current Compensator : Gain  Gain=Kffpv_i
  Current Compensator1 : Gain  Gain=Kffpv_i
  Damping (d)1 : Gain  Gain=Kpvp_v1
  Damping (q)1 : Gain  Gain=Kpvp_v1
  Demux : Demux  Outputs=2
  Demux2 : Demux  Outputs=2
  Demux3 : Demux  Outputs=2
  Discrete-Time Integrator : DiscreteIntegrator  SampleTime=T_s_cont  ICPrevOutput=DiscIntNeverNeededParam  ICPrevScaledInput=DiscIntNeverNeededParam
  Discrete-Time Integrator1 : DiscreteIntegrator  SampleTime=T_s_cont  ICPrevOutput=DiscIntNeverNeededParam  ICPrevScaledInput=DiscIntNeverNeededParam
  Eg_d * (wCf) : Product  RndMeth=Zero
  "Eg_q * (wCf) " : Product  RndMeth=Zero
  Filter capacitance : Gain  Gain=C_f
  G lowpass5 : DiscreteStateSpace  A=G_lowpass_disc_1khz.A  B=G_lowpass_disc_1khz.B  C=G_lowpass_disc_1khz.C  D=G_lowpass_disc_1khz.D  SampleTime=T_s_cont
  Integration Time : Gain  Gain=Kpvi_v1
  Integration Time1 : Gain  Gain=Kpvi_v1
  Is_0* : Constant  Value=0  SampleTime=T_s_cont
  Mux : Mux  Inputs=3
  Scope : Scope  NumInputPorts=2
  Selector : Selector  InputPortWidth=3  IndexOptions=Index vector (dialog)  Indices=[1 2]  OutputSizes=1
  Selector1 : Selector  InputPortWidth=3  IndexOptions=Index vector (dialog)  Indices=[1 2]  OutputSizes=1
  Selector2 : Selector  InputPortWidth=3  IndexOptions=Index vector (dialog)  Indices=[1 2]  OutputSizes=1
  Sum : Sum  Inputs=|+-
  Sum1 : Sum  Inputs=|++
  Sum2 : Sum  Inputs=|+-
  Sum3 : Sum  Inputs=|++
  Sum4 : Sum  Inputs=|++
  Sum5 : Sum  Inputs=++|
  Sum6 : Sum  Inputs=-+|
  Sum7 : Sum  Inputs=++|
  i_s_ref_dq0 : Outport  VectorParamsAs1DForOutWhenUnconnected=off
  wires:
  Is_0*/1 -> Mux/3
  w/1 -> Filter capacitance/1
  Integration Time1/1 -> Discrete-Time Integrator1/1
  Discrete-Time Integrator1/1 -> Sum4/1
  Eg_d * (wCf)/1 -> Sum5/1  "Is_f"
  Sum7/1 -> Mux/2  "Is_q*"
  Sum2/1 -> Sum3/1  "Is_d'"
  Current Compensator/1 -> Sum3/2
  Current Compensator1/1 -> Sum7/1
  "Eg_q * (wCf) "/1 -> Sum2/2  "Is_f"
  Filter capacitance/1 -> "Eg_q * (wCf) "/2, Eg_d * (wCf)/2
  Sum1/1 -> Sum2/1  "Is_d\""
  Sum5/1 -> Sum7/2  "Is_q'"
  Discrete-Time Integrator/1 -> Sum1/1
  Integration Time/1 -> Discrete-Time Integrator/1
  Sum3/1 -> Mux/1  "Is_d*"
  Sum4/1 -> Sum5/2  "Is_q\""
  Selector/1 -> Demux3/1
  Selector1/1 -> Demux/1
  Selector2/1 -> Demux2/1
  Mux/1 -> i_s_ref_dq0/1
  Sum/1 -> Damping (d)1/1, Integration Time/1
  Sum6/1 -> Damping (q)1/1, Integration Time1/1
  Demux/1 -> [vd_ref]  "Eg_d*"
  Demux/2 -> [vq_ref]  "Eg_q*"
  Demux3/1 -> Scope/2, [vd], Scope/1  "Eg_d*"
  Demux3/2 -> [vq]  "Eg_q*"
  [vd_ref] -> Sum/1
  [vq_ref] -> Sum6/2
  [vd] -> Sum/2
  [vq] -> Sum6/1
  Damping (q)1/1 -> Sum4/2  "Is_q\""
  Demux2/1 -> [id]  "Ig_d"
  [id] -> Current Compensator/1
  [iq] -> Current Compensator1/1
  Damping (d)1/1 -> Sum1/2  "Is_d\""
  [vd] -> Eg_d * (wCf)/1
  [vq] -> "Eg_q * (wCf) "/1
  v_ref_dq0/1 -> Selector1/1
  v_dq0/1 -> Selector/1
  i_dq0/1 -> Selector2/1
  Demux2/2 -> [iq]  "yes lowpass"

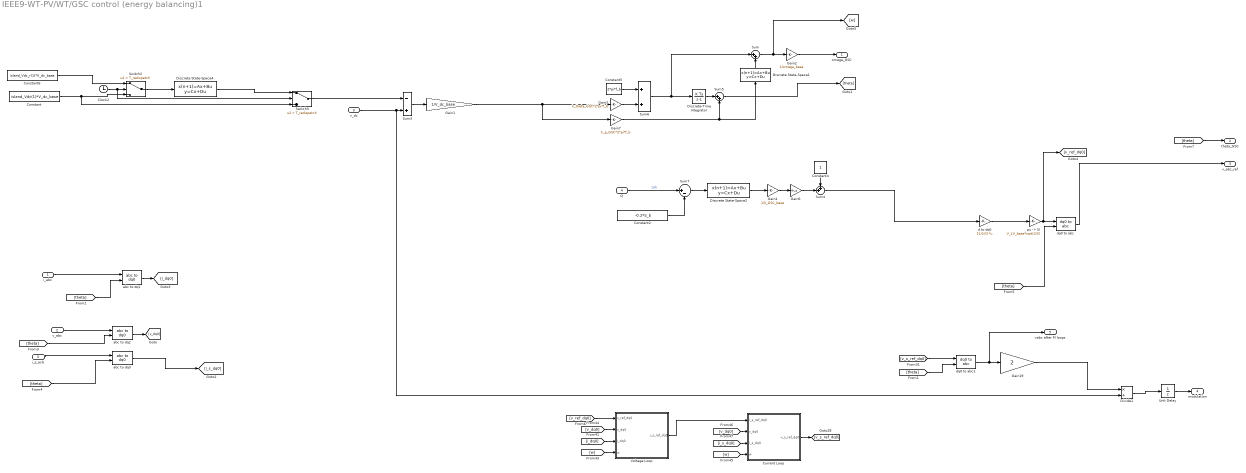
== system IEEE9-WT-PV/WT/GSC control (energy balancing)1 ==
  i_abc : Inport
  v_abc : Inport  Port=2
  v_dc : Inport  Port=3
  Q : Inport  Port=4
  i_s_acb : Inport  Port=5
  Clock2 : Clock
  Constant : Constant  Value=island_Vdc(1)*V_dc_base  SampleTime=T_s_cont
  Constant2 : Constant  Value=-0.2*S_b  SampleTime=T_s_cont
  Constant4 : Constant  SampleTime=T_s_cont
  Constant5 : Constant  Value=2*pi*f_b  SampleTime=T_s_cont
  Constant6 : Constant  Value=island_Vdc_r(1)*V_dc_base  SampleTime=T_s_cont
  Current Loop : Subsystem
  Discrete State-Space1 : DiscreteStateSpace  A=G_diff.A  B=G_diff.B  C=G_diff.C  D=G_diff.D  SampleTime=T_s_cont
  Discrete State-Space2 : DiscreteStateSpace  A=G_lowpass_disc.A  B=G_lowpass_disc.B  C=G_lowpass_disc.C  D=G_lowpass_disc.D  SampleTime=T_s_cont
  Discrete State-Space4 : DiscreteStateSpace  A=G_setpoint_lowpass_disc.A  B=G_setpoint_lowpass_disc.B  C=G_setpoint_lowpass_disc.C  D=G_setpoint_lowpass_disc.D  SampleTime=T_s_cont
  Discrete-Time Integrator : DiscreteIntegrator  InitialCondition=GSC_theta0  SampleTime=T_s_cont  ICPrevOutput=DiscIntNeverNeededParam  ICPrevScaledInput=DiscIntNeverNeededParam
  Divide1 : Product  Inputs=*/
  Gain1 : Gain  Gain=1/V_dc_base
  Gain19 : Gain  Gain=2
  Gain2 : Gain  Gain=1/omega_base
  Gain3 : Gain  Gain=k_theta_GSC*2*pi*f_b
  Gain4 : Gain  Gain=1/S_GSC_base
  Gain6 : Gain  Gain=fdr_q
  Gain7 : Gain  Gain=k_p_GSC*2*pi*f_b
  Sum : Sum  Inputs=|++
  Sum3 : Sum  Inputs=-+
  Sum4 : Sum  Inputs=++|
  Sum5 : Sum  Inputs=|++
  Sum6 : Sum
  Sum7 : Sum  Inputs=|+-
  Switch2 : Switch  Criteria=u2 > Threshold  Threshold=T_redispatch  SaturateOnIntegerOverflow=off  InputSameDT=off
  Switch3 : Switch  Criteria=u2 > Threshold  Threshold=T_redispatch  SaturateOnIntegerOverflow=off  InputSameDT=off
  Unit Delay : UnitDelay  SampleTime=T_s_sim  HasFrameUpgradeWarning=on
  Voltage Loop : Subsystem
  abc to dq1 : spsabctodq0Lib/abc to dq0  Alignment=90 degrees behind phase A axis
  abc to dq2 : spsabctodq0Lib/abc to dq0  Alignment=90 degrees behind phase A axis
  abc to dq3 : spsabctodq0Lib/abc to dq0  Alignment=90 degrees behind phase A axis
  d to dq0 : Gain  Gain=[1;0;0]  Multiplication=Matrix(K*u) (u vector)
  dq0 to abc : spsdq0toabcLib/dq0 to abc  Alignment=90 degrees behind phase A axis
  dq0 to abc1 : spsdq0toabcLib/dq0 to abc  Alignment=90 degrees behind phase A axis
  "pu -> SI" : Gain  Gain=V_LV_base*sqrt(2/3)
  omega_GSC : Outport
  theta_GSC : Outport  Port=2
  v_abc_ref : Outport  Port=3
  modulation : Outport  Port=4
  vabc after PI loops : Outport  Port=5
  wires:
  Sum3/1 -> Gain1/1
  i_abc/1 -> abc to dq1/1
  abc to dq1/1 -> [i_dq0]
  Constant4/1 -> Sum4/1
  Gain4/1 -> Gain6/1
  "pu -> SI"/1 -> [v_ref_dq0], dq0 to abc/1
  dq0 to abc/1 -> v_abc_ref/1
  Gain3/1 -> Sum6/2
  Discrete-Time Integrator/1 -> Sum5/1
  Constant5/1 -> Sum6/1
  Gain7/1 -> Sum5/2, Discrete State-Space1/1
  Sum6/1 -> Sum/1, Discrete-Time Integrator/1
  Gain2/1 -> omega_GSC/1
  Sum/1 -> [w], Gain2/1
  Discrete State-Space1/1 -> Sum/2
  Unit Delay/1 -> modulation/1
  Gain6/1 -> Sum4/2
  d to dq0/1 -> "pu -> SI"/1
  Sum4/1 -> d to dq0/1
  v_abc/1 -> abc to dq2/1
  abc to dq2/1 -> [v_dq0]
  [i_dq0] -> Voltage Loop/3(i_dq0)
  [v_dq0] -> Voltage Loop/2(v_dq0)
  [i_s_dq0] -> Current Loop/3(i_s_dq0)
  Gain19/1 -> Divide1/1
  [v_dq0] -> Current Loop/2(v_dq0)
  [v_s_ref_dq0] -> dq0 to abc1/1
  [w] -> Current Loop/4(w)
  Voltage Loop/1(i_s_ref_dq0) -> Current Loop/1(i_s_ref_dq0)
  dq0 to abc1/1 -> vabc after PI loops/1, Gain19/1
  [w] -> Voltage Loop/4(w)
  Current Loop/1(v_s_ref_dq0) -> [v_s_ref_dq0]
  i_s_acb/1 -> abc to dq3/1
  abc to dq3/1 -> [i_s_dq0]
  Sum5/1 -> [theta]
  [theta] -> dq0 to abc1/2
  [theta] -> abc to dq1/2
  [theta] -> abc to dq2/2
  [theta] -> abc to dq3/2
  [theta] -> dq0 to abc/2
  [v_ref_dq0] -> Voltage Loop/1(v_ref_dq0)
  v_dc/1 -> Divide1/2, Sum3/2
  Divide1/1 -> Unit Delay/1
  [theta] -> theta_GSC/1
  Sum7/1 -> Discrete State-Space2/1
  Switch2/1 -> Discrete State-Space4/1
  Constant/1 -> Switch2/3, Switch3/3
  Clock2/1 -> Switch3/2, Switch2/2
  Constant6/1 -> Switch2/1
  Discrete State-Space4/1 -> Switch3/1
  Switch3/1 -> Sum3/1
  Constant2/1 -> Sum7/2
  Discrete State-Space2/1 -> Gain4/1
  Q/1 -> Sum7/1  "zoh"
  Gain1/1 -> Gain7/1, Gain3/1

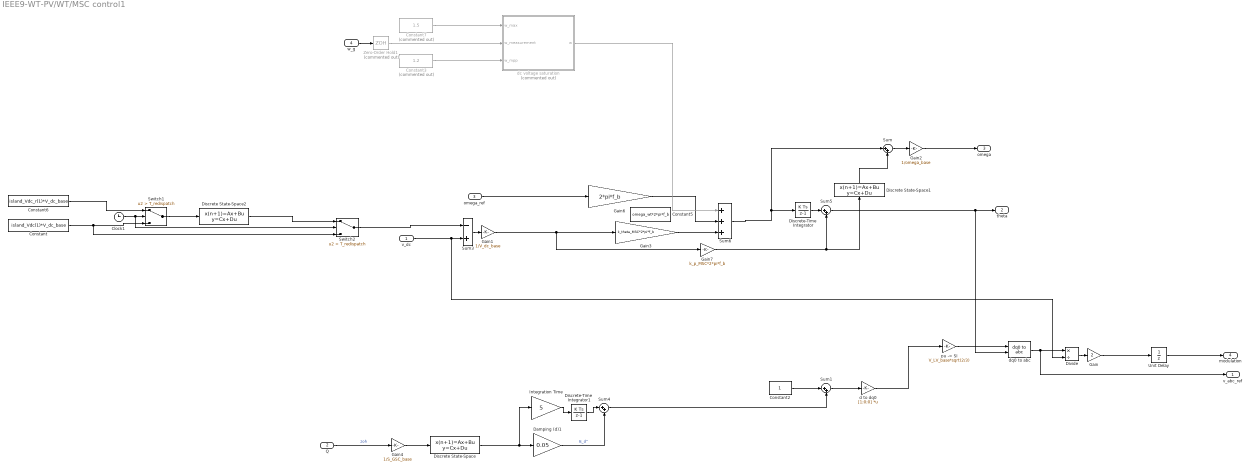
== system IEEE9-WT-PV/WT/MSC control1 ==
  v_dc : Inport
  Q : Inport  Port=2
  omega_ref : Inport  Port=3
  w_g : Inport  Port=4
  Clock1 : Clock
  Constant : Constant  Value=island_Vdc(1)*V_dc_base  SampleTime=T_s_cont
  Constant2 : Constant  SampleTime=T_s_cont
  Constant3 : Constant  Commented=on  Value=1.2  SampleTime=T_s_cont
  Constant5 : Constant  Value=omega_wt*2*pi*f_b  SampleTime=T_s_cont
  Constant6 : Constant  Value=island_Vdc_r(1)*V_dc_base  SampleTime=T_s_cont
  Constant7 : Constant  Commented=on  Value=1.5  SampleTime=T_s_cont
  Damping (d)1 : Gain  Gain=0.05
  Discrete State-Space : DiscreteStateSpace  A=G_lowpass_disc.A  B=G_lowpass_disc.B  C=G_lowpass_disc.C  D=G_lowpass_disc.D  SampleTime=T_s_cont
  Discrete State-Space1 : DiscreteStateSpace  A=G_diff.A  B=G_diff.B  C=G_diff.C  D=G_diff.D  SampleTime=T_s_cont
  Discrete State-Space2 : DiscreteStateSpace  A=G_setpoint_lowpass_disc.A  B=G_setpoint_lowpass_disc.B  C=G_setpoint_lowpass_disc.C  D=G_setpoint_lowpass_disc.D  SampleTime=T_s_cont
  Discrete-Time Integrator : DiscreteIntegrator  InitialCondition=RSC_theta0+T_s_cont/2*omega_wt*2*pi*f_b  SampleTime=T_s_cont  ICPrevOutput=DiscIntNeverNeededParam  ICPrevScaledInput=DiscIntNeverNeededParam
  Discrete-Time Integrator1 : DiscreteIntegrator  SampleTime=T_s_cont  ICPrevOutput=DiscIntNeverNeededParam  ICPrevScaledInput=DiscIntNeverNeededParam
  Divide : Product  Inputs=*/
  Gain : Gain  Gain=2
  Gain1 : Gain  Gain=1/V_dc_base
  Gain2 : Gain  Gain=1/omega_base
  Gain3 : Gain  Gain=k_theta_MSC*2*pi*f_b
  Gain4 : Gain  Gain=1/S_GSC_base
  Gain6 : Gain  Gain=2*pi*f_b
  Gain7 : Gain  Gain=k_p_MSC*2*pi*f_b
  Integration Time : Gain  Gain=5
  Sum{,1,4..5} (4 alike) : Sum  Inputs=|++
  Sum3 : Sum  Inputs=-+
  Sum6 : Sum  Inputs=+++
  Switch1 : Switch  Criteria=u2 > Threshold  Threshold=T_redispatch  SaturateOnIntegerOverflow=off  InputSameDT=off
  Switch2 : Switch  Criteria=u2 > Threshold  Threshold=T_redispatch  SaturateOnIntegerOverflow=off  InputSameDT=off
  Unit Delay : UnitDelay  SampleTime=T_s_sim  HasFrameUpgradeWarning=on
  Zero-Order Hold1 : ZeroOrderHold  Commented=on  SampleTime=T_s_cont
  d to dq0 : Gain  Gain=[1;0;0]  Multiplication=Matrix(K*u) (u vector)
  dc voltage saturation : Subsystem  Commented=on
  dq0 to abc : spsdq0toabcLib/dq0 to abc  Alignment=90 degrees behind phase A axis
  "pu -> SI" : Gain  Gain=V_LV_base*sqrt(2/3)
  v_abc_ref : Outport
  theta : Outport  Port=2
  omega : Outport  Port=3
  modulation : Outport  Port=4
  wires:
  Sum4/1 -> Sum1/2
  Gain6/1 -> Sum6/2
  Gain3/1 -> Sum6/3
  w_g/1 -> Zero-Order Hold1/1
  Constant7/1 -> dc voltage saturation/1(w_max)
  Zero-Order Hold1/1 -> dc voltage saturation/2(w_measurement)
  Constant3/1 -> dc voltage saturation/3(w_mpp)
  omega_ref/1 -> Gain6/1
  Switch2/1 -> Sum3/1
  Discrete State-Space2/1 -> Switch2/1
  Constant/1 -> Switch2/3, Switch1/3
  Clock1/1 -> Switch1/2, Switch2/2
  Constant6/1 -> Switch1/1
  Switch1/1 -> Discrete State-Space2/1
  Unit Delay/1 -> modulation/1
  d to dq0/1 -> "pu -> SI"/1
  Sum6/1 -> Discrete-Time Integrator/1, Sum/1
  Sum5/1 -> theta/1, dq0 to abc/2
  Divide/1 -> Gain/1
  Discrete State-Space1/1 -> Sum/2
  Discrete-Time Integrator/1 -> Sum5/1
  Sum/1 -> Gain2/1
  Gain7/1 -> Discrete State-Space1/1, Sum5/2
  Sum3/1 -> Gain1/1
  v_dc/1 -> Divide/2, Sum3/2
  Gain2/1 -> omega/1
  Gain4/1 -> Discrete State-Space/1
  Gain/1 -> Unit Delay/1
  Sum1/1 -> d to dq0/1
  Constant2/1 -> Sum1/1
  "pu -> SI"/1 -> dq0 to abc/1
  dq0 to abc/1 -> Divide/1, v_abc_ref/1
  Gain1/1 -> Gain3/1, Gain7/1
  Q/1 -> Gain4/1  "zoh"
  dc voltage saturation/1(w) -> Sum6/1
  Discrete-Time Integrator1/1 -> Sum4/1
  Damping (d)1/1 -> Sum4/2  "Is_d\""
  Integration Time/1 -> Discrete-Time Integrator1/1
  Discrete State-Space/1 -> Integration Time/1, Damping (d)1/1

== system IEEE9-WT-PV/WT/pitch angle controller ==
  wg : Inport
  max : Inport  Port=2
  omega_ref : Inport  Port=3
  Constant : Constant  Value=beta_0  SampleTime=T_s_cont
  Constant5 : Constant  Value=1.2  SampleTime=T_s_cont
  Damping (d)1 : Gain  Gain=PI_pitch.Ka
  Damping (d)2 : Gain  Gain=PI_pitch.Ka
  Discrete-Time Integrator : DiscreteIntegrator  SampleTime=T_s_cont  ICPrevOutput=DiscIntNeverNeededParam  ICPrevScaledInput=DiscIntNeverNeededParam
  Discrete-Time Integrator1 : DiscreteIntegrator  InitialCondition=beta_0  SampleTime=T_s_cont  LimitOutput=on  UpperSaturationLimit=27  LowerSaturationLimit=0  ICPrevOutput=DiscIntNeverNeededParam  ICPrevScaledInput=DiscIntNeverNeededParam
  Discrete-Time Integrator2 : DiscreteIntegrator  SampleTime=T_s_cont  ICPrevOutput=DiscIntNeverNeededParam  ICPrevScaledInput=DiscIntNeverNeededParam
  Gain : Gain  Gain=Kp_beta
  Integration Time : Gain  Gain=PI_pitch.Tr
  Integration Time1 : Gain  Gain=PI_pitch.Tr
  Saturation : Saturate  UpperLimit=27  LowerLimit=0
  Saturation1 : Saturate  UpperLimit=27  LowerLimit=0
  Sum : Sum  Inputs=++-
  Sum1 : Sum  Inputs=|+-
  Sum2 : Sum  Inputs=-+|
  Sum3 : Sum  Inputs=|+-
  Sum4 : Sum  Inputs=|+-
  Sum5 : Sum  Inputs=++|
  Sum6 : Sum  Inputs=|++
  Sum7 : Sum  Inputs=|++
  Unit Delay : UnitDelay  SampleTime=T_s_sim  HasFrameUpgradeWarning=on
  rate limiter : Saturate  UpperLimit=10  LowerLimit=-10
  time constant : Gain  Gain=1/T_pitch_servo
  pitch : Outport
  wires:
  wg/1 -> Sum4/1, Sum1/1, Sum3/2
  max/1 -> Sum1/2
  Sum/1 -> time constant/1
  Discrete-Time Integrator1/1 -> Sum/3, Unit Delay/1
  time constant/1 -> rate limiter/1
  rate limiter/1 -> Discrete-Time Integrator1/1
  Constant/1 -> Sum2/2
  Constant5/1 -> Sum3/1
  Sum4/1 -> Gain/1
  Sum2/1 -> Sum5/2
  Sum5/1 -> Sum/1
  Gain/1 -> Sum5/1
  Unit Delay/1 -> pitch/1
  omega_ref/1 -> Sum4/2
  Sum6/1 -> Saturation/1
  Saturation1/1 -> Sum/2
  Sum3/1 -> Integration Time/1, Damping (d)1/1
  Discrete-Time Integrator/1 -> Sum6/1
  Damping (d)1/1 -> Sum6/2  "Is_d\""
  Integration Time/1 -> Discrete-Time Integrator/1
  Saturation/1 -> Sum2/1
  Sum7/1 -> Saturation1/1
  Discrete-Time Integrator2/1 -> Sum7/1
  Damping (d)2/1 -> Sum7/2  "Is_d\""
  Integration Time1/1 -> Discrete-Time Integrator2/1
  Sum1/1 -> Damping (d)2/1, Integration Time1/1

== system IEEE9-WT-PV/VSC 2/PV parsitic1/Subsystem1 ==
  note: Idiod
  note: Vd
  Vpv : Inport
  Add : Sum  Inputs=+-
  Constant2 : Constant  SampleTime=T_s_sim
  Gain : Gain  Gain=1/VT_total1
  Gain3 : Gain  Gain=I0_total1
  Math Function : Math
  Saturation2 : Saturate  UpperLimit=Ipv_scmax1  LowerLimit=0
  Scope1 : Scope  NumInputPorts=3
  Scope2 : Scope  NumInputPorts=2
  Unit Delay : UnitDelay  SampleTime=T_s_sim  HasFrameUpgradeWarning=on
  Idiod : Outport  VectorParamsAs1DForOutWhenUnconnected=off
  wires:
  Gain3/1 -> Scope1/2, Saturation2/1
  Math Function/1 -> Scope2/1, Add/1
  Constant2/1 -> Add/2
  Gain/1 -> Math Function/1
  Add/1 -> Scope1/1, Gain3/1
  Vpv/1 -> Gain/1
  Saturation2/1 -> Scope1/3, Unit Delay/1
  Unit Delay/1 -> Idiod/1

== system IEEE9-WT-PV/VSC 2/VSC (energy balancing)1/dc voltage saturation ==
  V_open_circuit : Inport
  Vdc_measurement : Inport  Port=2
  V_mpp : Inport  Port=3
  Discrete-Time Integrator1 : DiscreteIntegrator  SampleTime=T_s_cont  LimitOutput=on  UpperSaturationLimit=0  ICPrevOutput=DiscIntNeverNeededParam  ICPrevScaledInput=DiscIntNeverNeededParam
  Discrete-Time Integrator2 : DiscreteIntegrator  SampleTime=T_s_cont  LimitOutput=on  LowerSaturationLimit=0  ICPrevOutput=DiscIntNeverNeededParam  ICPrevScaledInput=DiscIntNeverNeededParam
  Gain1 : Gain  Gain=0.63
  Gain10 : Gain  Gain=w_b/Vdc_n
  Gain2 : Gain  Gain=0.09
  Gain3 : Gain  Gain=w_b/Vdc_n
  Gain4 : Gain  Gain=1/Vdc_n
  Gain5 : Gain  Gain=0.71
  Gain7 : Gain  Gain=0.03
  Saturation1 : Saturate  UpperLimit=inf  LowerLimit=0
  Saturation2 : Saturate  UpperLimit=0  LowerLimit=-inf
  Scope2 : Scope
  Scope3 : Scope
  Sum10 : Sum  Inputs=|++
  Sum11 : Sum  Inputs=|++
  Sum12 : Sum  Inputs=+-
  Sum17 : Sum  Inputs=+|+
  Sum8 : Sum  Inputs=-+
  w : Outport
  wires:
  V_mpp/1 -> Sum12/2
  Sum17/1 -> w/1
  Gain2/1 -> Discrete-Time Integrator2/1
  Discrete-Time Integrator1/1 -> Sum11/2
  Sum8/1 -> Gain3/1
  Gain7/1 -> Saturation1/1
  Gain1/1 -> Discrete-Time Integrator1/1
  Gain10/1 -> Scope2/1, Gain1/1, Gain5/1
  Sum10/1 -> Sum17/1
  Saturation1/1 -> Sum10/1
  Discrete-Time Integrator2/1 -> Sum10/2
  Gain5/1 -> Saturation2/1
  Vdc_measurement/1 -> Sum8/2, Sum12/1
  Sum12/1 -> Gain10/1, Gain4/1
  Saturation2/1 -> Sum11/1
  Gain3/1 -> Gain7/1, Gain2/1
  V_open_circuit/1 -> Sum8/1
  Sum11/1 -> Sum17/2
  Gain4/1 -> Scope3/1

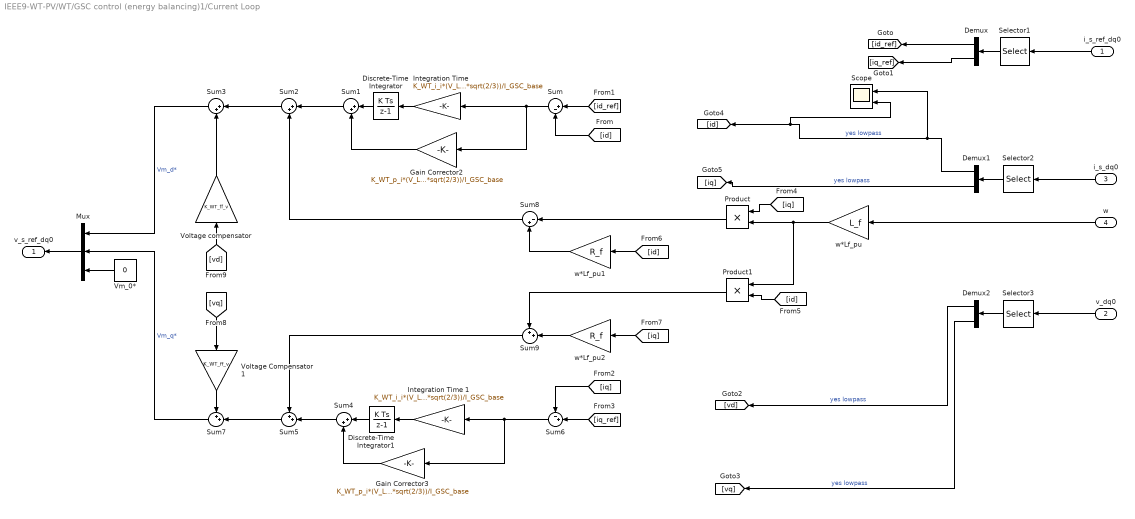
== system IEEE9-WT-PV/WT/GSC control (energy balancing)1/Current Loop ==
  i_s_ref_dq0 : Inport
  v_dq0 : Inport  Port=2
  i_s_dq0 : Inport  Port=3
  w : Inport  Port=4
  Demux : Demux  Outputs=2
  Demux1 : Demux  Outputs=2
  Demux2 : Demux  Outputs=2
  Discrete-Time Integrator : DiscreteIntegrator  SampleTime=T_s_cont  ICPrevOutput=DiscIntNeverNeededParam  ICPrevScaledInput=DiscIntNeverNeededParam
  Discrete-Time Integrator1 : DiscreteIntegrator  SampleTime=T_s_cont  ICPrevOutput=DiscIntNeverNeededParam  ICPrevScaledInput=DiscIntNeverNeededParam
  Gain Corrector2 : Gain  Gain=K_WT_p_i*(V_LV_base*sqrt(2/3))/I_GSC_base
  Gain Corrector3 : Gain  Gain=K_WT_p_i*(V_LV_base*sqrt(2/3))/I_GSC_base
  Integration Time : Gain  Gain=K_WT_i_i*(V_LV_base*sqrt(2/3))/I_GSC_base
  Integration Time 1 : Gain  Gain=K_WT_i_i*(V_LV_base*sqrt(2/3))/I_GSC_base
  Mux : Mux  Inputs=3
  Product : Product  RndMeth=Zero
  Product1 : Product  RndMeth=Zero
  Scope : Scope  NumInputPorts=2
  Selector1 : Selector  InputPortWidth=3  IndexOptions=Index vector (dialog)  Indices=[1 2]  OutputSizes=1
  Selector2 : Selector  InputPortWidth=3  IndexOptions=Index vector (dialog)  Indices=[1 2]  OutputSizes=1
  Selector3 : Selector  InputPortWidth=3  IndexOptions=Index vector (dialog)  Indices=[1 2]  OutputSizes=1
  Sum : Sum  Inputs=|+-
  Sum{1..4} (4 alike) : Sum  Inputs=|++
  Sum5 : Sum  Inputs=++|
  Sum6 : Sum  Inputs=-+|
  Sum7 : Sum  Inputs=++|
  Sum8 : Sum  Inputs=|-+
  Sum9 : Sum  Inputs=++|
  Vm_0* : Constant  Value=0  SampleTime=T_s_cont
  Voltage Compensator 1 : Gain  Gain=K_WT_ff_v
  Voltage compensator : Gain  Gain=K_WT_ff_v
  w*Lf_pu : Gain  Gain=L_f
  w*Lf_pu1 : Gain  Gain=R_f
  w*Lf_pu2 : Gain  Gain=R_f
  v_s_ref_dq0 : Outport  VectorParamsAs1DForOutWhenUnconnected=off
  wires:
  Integration Time 1/1 -> Discrete-Time Integrator1/1
  Integration Time/1 -> Discrete-Time Integrator/1
  Sum5/1 -> Sum7/2
  Sum3/1 -> Mux/1  "Vm_d*"
  Sum7/1 -> Mux/2  "Vm_q*"
  Voltage Compensator 1/1 -> Sum7/1
  w*Lf_pu/1 -> Product1/1, Product/2
  i_s_ref_dq0/1 -> Selector1/1
  Discrete-Time Integrator1/1 -> Sum4/1
  Voltage compensator/1 -> Sum3/2
  Sum2/1 -> Sum3/1
  Selector1/1 -> Demux/1
  Sum1/1 -> Sum2/1
  w/1 -> w*Lf_pu/1
  Mux/1 -> v_s_ref_dq0/1
  Selector2/1 -> Demux1/1
  Selector3/1 -> Demux2/1
  Vm_0*/1 -> Mux/3
  Discrete-Time Integrator/1 -> Sum1/1
  Sum4/1 -> Sum5/2
  Sum/1 -> Integration Time/1, Gain Corrector2/1
  Sum6/1 -> Integration Time 1/1, Gain Corrector3/1
  Demux/1 -> [id_ref]
  Demux/2 -> [iq_ref]
  [id] -> Sum/2
  [id_ref] -> Sum/1
  [iq_ref] -> Sum6/2
  [iq] -> Sum6/1
  Gain Corrector2/1 -> Sum1/2
  Gain Corrector3/1 -> Sum4/2
  [iq] -> Product/1
  [id] -> Product1/2
  Product/1 -> Sum8/1
  [id] -> w*Lf_pu1/1
  w*Lf_pu1/1 -> Sum8/2
  Sum8/1 -> Sum2/2
  Product1/1 -> Sum9/1
  [iq] -> w*Lf_pu2/1
  w*Lf_pu2/1 -> Sum9/2
  Sum9/1 -> Sum5/1
  [vq] -> Voltage Compensator 1/1
  [vd] -> Voltage compensator/1
  v_dq0/1 -> Selector3/1
  i_s_dq0/1 -> Selector2/1
  Demux1/1 -> Scope/2, [id], Scope/1  "yes lowpass"
  Demux1/2 -> [iq]  "yes lowpass"
  Demux2/1 -> [vd]  "yes lowpass"
  Demux2/2 -> [vq]  "yes lowpass"
